simulink model "controle_kanayama"  (R2018a)
settings: Solver=VariableStepAuto  StartTime=0.0  StopTime=7  RelTol=1e-3
values from neighbouring files (symbols this model uses):
  KIm = Pm*KPm    (= 0.759312111233)    [LineFollower.m]    (also in malha_fechada.m)
  Km = 455.5    [LineFollower.m]    (also in malha_aberta.m; malha_fechada.m)
  KPm = 4/(Km*ts_m)    (= 0.0585437248445)    [LineFollower.m]    (also in malha_fechada.m)
  Kteta = 2*qsi*sqrt(Ky)    [LineFollower.m]
  Kx = 4/Ts_x    (= 80)    [LineFollower.m]
  Ky = (wn/v_r)^2    (= 6400)    [LineFollower.m]
  l = 69e-3    (= 0.069)    [LineFollower.m]    (also in malha_aberta.m; malha_fechada.m)
  Pm = 12.97    [LineFollower.m]    (also in malha_aberta.m; malha_fechada.m)
  Qr = [v_r; w_r]    [LineFollower.m]
  r = 16e-3    (= 0.016)    [LineFollower.m]    (also in kinematic_model.m; malha_aberta.m; malha_fechada.m)
libraries: simulink x6
settings Model: Creator=bruno  LastModifiedBy=bruno

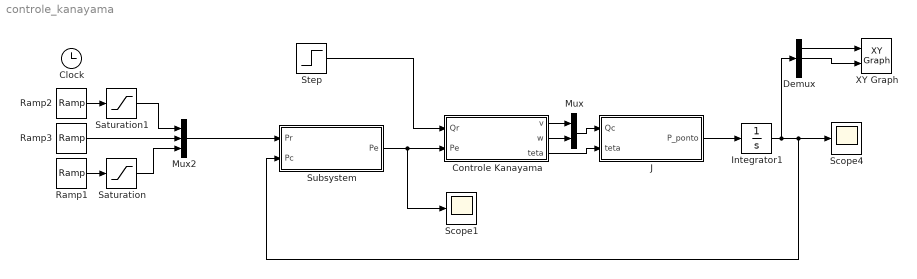
== system controle_kanayama ==
  Clock : Clock
  Controle Kanayama : Subsystem
  Demux : Demux  Outputs=3
  Integrator1 : Integrator
  J : Subsystem
  Mux : Mux  Inputs=2
  Mux2 : Mux  Inputs=3
  Ramp1 : simulink/Sources/Ramp  slope=5  start=0  InitialOutput=0
  Ramp2 : simulink/Sources/Ramp  slope=1  start=0  InitialOutput=0
  Ramp3 : simulink/Sources/Ramp  slope=0  start=0  InitialOutput=0
  Saturation : Saturate  UpperLimit=0
  Saturation1 : Saturate  UpperLimit=1
  Scope1 : Scope
  Scope4 : Scope
  Step : Step  Time=0  After=Qr  SampleTime=0
  Subsystem : Subsystem
  XY Graph : simulink/Sinks/XY Graph  xmin=0  xmax=6  ymin=-0.06  ymax=0.06  st=-1
  wires:
  Integrator1/1 -> Demux/1, Scope4/1, Subsystem/2(Pc)
  Subsystem/1(Pe) -> Scope1/1, Controle Kanayama/2(Pe)
  J/1(P_ponto) -> Integrator1/1
  Mux/1 -> J/1(Qc)
  Controle Kanayama/1(v) -> Mux/1
  Controle Kanayama/2(w) -> Mux/2
  Controle Kanayama/3(teta) -> J/2(teta)
  Step/1 -> Controle Kanayama/1(Qr)
  Ramp3/1 -> Mux2/2
  Ramp1/1 -> Saturation/1
  Saturation/1 -> Mux2/3
  Demux/1 -> XY Graph/1
  Demux/2 -> XY Graph/2
  Ramp2/1 -> Saturation1/1
  Saturation1/1 -> Mux2/1
  Mux2/1 -> Subsystem/1(Pr)

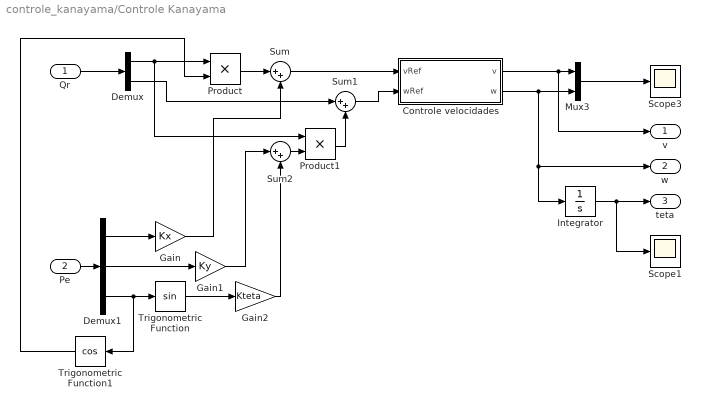
== system controle_kanayama/Controle Kanayama ==
  Qr : Inport
  Pe : Inport  Port=2
  Controle velocidades : Subsystem
  Demux : Demux  Outputs=2
  Demux1 : Demux  Outputs=3
  Gain : Gain  Gain=Kx
  Gain1 : Gain  Gain=Ky
  Gain2 : Gain  Gain=Kteta
  Integrator : Integrator
  Mux3 : Mux  Inputs=2
  Product : Product
  Product1 : Product
  Scope1 : Scope
  Scope3 : Scope
  Sum : Sum  Inputs=|++
  Sum1 : Sum  Inputs=|++
  Sum2 : Sum  Inputs=|++
  Trigonometric Function : Trigonometry
  Trigonometric Function1 : Trigonometry  Operator=cos
  v : Outport
  w : Outport  Port=2
  teta : Outport  Port=3
  wires:
  Controle velocidades/2(w) -> Integrator/1, w/1, Mux3/2
  Controle velocidades/1(v) -> v/1, Mux3/1
  Mux3/1 -> Scope3/1
  Integrator/1 -> Scope1/1, teta/1
  Qr/1 -> Demux/1
  Pe/1 -> Demux1/1
  Demux/1 -> Product/1, Product1/1
  Trigonometric Function/1 -> Gain2/1
  Demux1/3 -> Trigonometric Function1/1, Trigonometric Function/1
  Product/1 -> Sum/1
  Sum/1 -> Controle velocidades/1(vRef)
  Demux1/1 -> Gain/1
  Gain/1 -> Sum/2
  Demux/2 -> Sum1/1
  Product1/1 -> Sum1/2
  Sum1/1 -> Controle velocidades/2(wRef)
  Sum2/1 -> Product1/2
  Demux1/2 -> Gain1/1
  Gain1/1 -> Sum2/1
  Gain2/1 -> Sum2/2
  Trigonometric Function1/1 -> Product/2

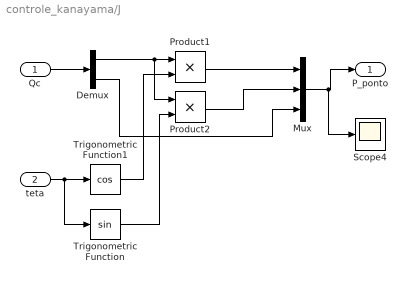
== system controle_kanayama/J ==
  Qc : Inport
  teta : Inport  Port=2
  Demux : Demux  Outputs=2
  Mux : Mux  Inputs=3
  Product1 : Product
  Product2 : Product
  Scope4 : Scope
  Trigonometric Function : Trigonometry
  Trigonometric Function1 : Trigonometry  Operator=cos
  P_ponto : Outport
  wires:
  Mux/1 -> Scope4/1, P_ponto/1
  Qc/1 -> Demux/1
  teta/1 -> Trigonometric Function/1, Trigonometric Function1/1
  Trigonometric Function1/1 -> Product1/2
  Demux/1 -> Product2/1, Product1/1
  Product1/1 -> Mux/1
  Trigonometric Function/1 -> Product2/2
  Product2/1 -> Mux/2
  Demux/2 -> Mux/3

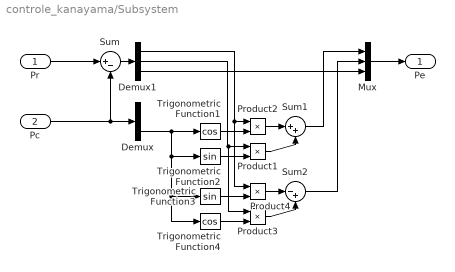
== system controle_kanayama/Subsystem ==
  Pr : Inport
  Pc : Inport  Port=2
  Demux : Demux  Outputs=3
  Demux1 : Demux  Outputs=3
  Mux : Mux  Inputs=3
  Product{1..4} (4 alike) : Product
  Sum : Sum  Inputs=|+-
  Sum1 : Sum  Inputs=|++
  Sum2 : Sum  Inputs=|-+
  Trigonometric Function1 : Trigonometry  Operator=cos
  Trigonometric Function2 : Trigonometry
  Trigonometric Function3 : Trigonometry
  Trigonometric Function4 : Trigonometry  Operator=cos
  Pe : Outport
  wires:
  Pr/1 -> Sum/1
  Pc/1 -> Demux/1, Sum/2
  Demux/3 -> Trigonometric Function4/1, Trigonometric Function3/1, Trigonometric Function2/1, Trigonometric Function1/1
  Sum/1 -> Demux1/1
  Trigonometric Function1/1 -> Product2/2
  Trigonometric Function2/1 -> Product1/2
  Demux1/1 -> Product4/1, Product2/1
  Demux1/2 -> Product3/1, Product1/1
  Product2/1 -> Sum1/1
  Product1/1 -> Sum1/2
  Mux/1 -> Pe/1
  Sum1/1 -> Mux/1
  Trigonometric Function3/1 -> Product4/2
  Product3/1 -> Sum2/2
  Trigonometric Function4/1 -> Product3/2
  Product4/1 -> Sum2/1
  Sum2/1 -> Mux/2
  Demux1/3 -> Mux/3

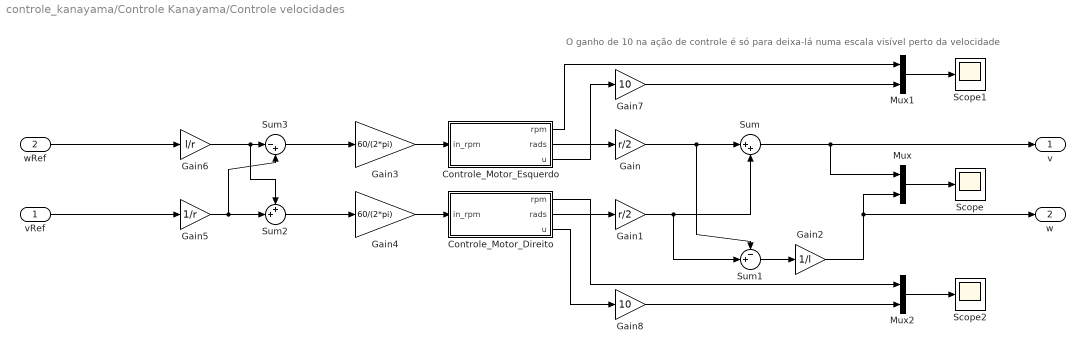
== system controle_kanayama/Controle Kanayama/Controle velocidades ==
  note: O ganho de 10 na ação de controle é só para deixa-lá numa escala visível perto da velocidade
  vRef : Inport
  wRef : Inport  Port=2
  Controle_Motor_Direito : Subsystem
  Controle_Motor_Esquerdo : Subsystem
  Gain : Gain  Gain=r/2
  Gain1 : Gain  Gain=r/2
  Gain2 : Gain  Gain=1/l
  Gain3 : Gain  Gain=60/(2*pi)
  Gain4 : Gain  Gain=60/(2*pi)
  Gain5 : Gain  Gain=1/r
  Gain6 : Gain  Gain=l/r
  Gain7 : Gain  Gain=10
  Gain8 : Gain  Gain=10
  Mux : Mux  Inputs=2
  Mux1 : Mux  Inputs=2
  Mux2 : Mux  Inputs=2
  Scope : Scope
  Scope1 : Scope
  Scope2 : Scope
  Sum : Sum  Inputs=|++
  Sum1 : Sum  Inputs=-+|
  Sum2 : Sum  Inputs=++|
  Sum3 : Sum  Inputs=|-+
  v : Outport
  w : Outport  Port=2
  wires:
  Sum2/1 -> Gain4/1
  vRef/1 -> Gain5/1
  Gain7/1 -> Mux1/2
  wRef/1 -> Gain6/1
  Gain2/1 -> w/1, Mux/2
  Gain1/1 -> Sum1/2, Sum/2
  Sum1/1 -> Gain2/1
  Controle_Motor_Direito/2(rads) -> Gain1/1
  Mux2/1 -> Scope2/1
  Gain3/1 -> Controle_Motor_Esquerdo/1(in_rpm)
  Mux/1 -> Scope/1
  Gain4/1 -> Controle_Motor_Direito/1(in_rpm)
  Gain/1 -> Sum1/1, Sum/1
  Gain5/1 -> Sum2/2, Sum3/2
  Mux1/1 -> Scope1/1
  Gain8/1 -> Mux2/2
  Controle_Motor_Esquerdo/3(u) -> Gain7/1
  Gain6/1 -> Sum2/1, Sum3/1
  Sum3/1 -> Gain3/1
  Controle_Motor_Esquerdo/1(rpm) -> Mux1/1
  Controle_Motor_Direito/3(u) -> Gain8/1
  Sum/1 -> v/1, Mux/1
  Controle_Motor_Direito/1(rpm) -> Mux2/1
  Controle_Motor_Esquerdo/2(rads) -> Gain/1

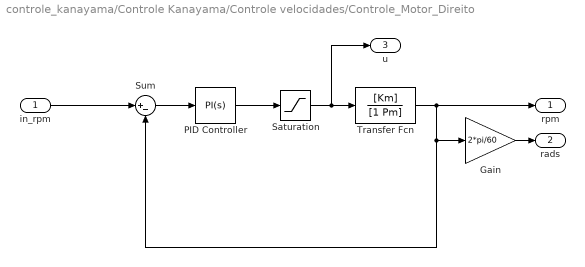
== system controle_kanayama/Controle Kanayama/Controle velocidades/Controle_Motor_Direito ==
  in_rpm : Inport
  Gain : Gain  Gain=2*pi/60
  PID Controller : simulink/Continuous/PID Controller  Controller=PI  TimeDomain=Continuous-time  SampleTime=-1  IntegratorMethod=Forward Euler  FilterMethod=Forward Euler  Form=Parallel  UseFilter=on  ControllerParametersSource=internal  P=KPm  I=KIm  D=0  N=0  InitialConditionSource=internal  InitialConditionForIntegrator=0  InitialConditionForFilter=0  ExternalReset=none  LimitOutput=off  UpperSaturationLimit=inf  LowerSaturationLimit=-inf  LinearizeAsGain=on  AntiWindupMode=none  Kb=1  TrackingMode=off  Kt=1  PParamMin=[]  PParamMax=[]  IParamMin=[]  IParamMax=[]  DParamMin=[]  DParamMax=[]  NParamMin=[]  NParamMax=[]  KbParamMin=[]  KbParamMax=[]  KtParamMin=[]  KtParamMax=[]  POutMin=[]  POutMax=[]  IOutMin=[]  IOutMax=[]  DOutMin=[]  DOutMax=[]  NOutMin=[]  NOutMax=[]  KbOutMin=[]  KbOutMax=[]  KtOutMin=[]  KtOutMax=[]  IntegratorOutMin=[]  IntegratorOutMax=[]  FilterOutMin=[]  FilterOutMax=[]  SumOutMin=[]  SumOutMax=[]  SumI1OutMin=[]  SumI1OutMax=[]  SumI2OutMin=[]  SumI2OutMax=[]  SumI3OutMin=[]  SumI3OutMax=[]  SumDOutMin=[]  SumDOutMax=[]  SaturationOutMin=[]  SaturationOutMax=[]  IntegratorContinuousStateAttributes=''  IntegratorStateMustResolveToSignalObject=off  IntegratorRTWStateStorageClass=Auto  FilterContinuousStateAttributes=''  FilterStateMustResolveToSignalObject=off  FilterRTWStateStorageClass=Auto  DifferentiatorICPrevScaledInput=0  DifferentiatorOutMin=[]  DifferentiatorOutMax=[]  FilterDiffOutCoefMin=[]  FilterDiffOutCoefMax=[]  SumDenOutMin=[]  SumDenOutMax=[]  SumNumOutMin=[]  SumNumOutMax=[]  ReciprocalOutMin=[]  ReciprocalOutMax=[]  DivideOutMin=[]  DivideOutMax=[]  TunerSelectOption=Transfer Function Based (PID Tuner App)
  Saturation : Saturate  UpperLimit=100  LowerLimit=-100
  Sum : Sum  Inputs=|+-
  Transfer Fcn : TransferFcn  Numerator=[Km]  Denominator=[1 Pm]
  rpm : Outport
  rads : Outport  Port=2
  u : Outport  Port=3
  wires:
  PID Controller/1 -> Saturation/1
  Transfer Fcn/1 -> rpm/1, Gain/1, Sum/2
  Saturation/1 -> u/1, Transfer Fcn/1
  Sum/1 -> PID Controller/1
  in_rpm/1 -> Sum/1
  Gain/1 -> rads/1

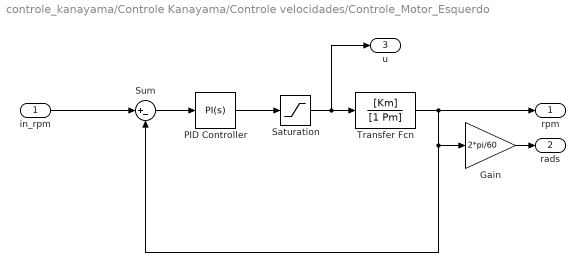
== system controle_kanayama/Controle Kanayama/Controle velocidades/Controle_Motor_Esquerdo ==
  in_rpm : Inport
  Gain : Gain  Gain=2*pi/60
  PID Controller : simulink/Continuous/PID Controller  Controller=PI  TimeDomain=Continuous-time  SampleTime=-1  IntegratorMethod=Forward Euler  FilterMethod=Forward Euler  Form=Parallel  UseFilter=on  ControllerParametersSource=internal  P=KPm  I=KIm  D=0  N=0  InitialConditionSource=internal  InitialConditionForIntegrator=0  InitialConditionForFilter=0  ExternalReset=none  LimitOutput=off  UpperSaturationLimit=inf  LowerSaturationLimit=-inf  LinearizeAsGain=on  AntiWindupMode=none  Kb=1  TrackingMode=off  Kt=1  PParamMin=[]  PParamMax=[]  IParamMin=[]  IParamMax=[]  DParamMin=[]  DParamMax=[]  NParamMin=[]  NParamMax=[]  KbParamMin=[]  KbParamMax=[]  KtParamMin=[]  KtParamMax=[]  POutMin=[]  POutMax=[]  IOutMin=[]  IOutMax=[]  DOutMin=[]  DOutMax=[]  NOutMin=[]  NOutMax=[]  KbOutMin=[]  KbOutMax=[]  KtOutMin=[]  KtOutMax=[]  IntegratorOutMin=[]  IntegratorOutMax=[]  FilterOutMin=[]  FilterOutMax=[]  SumOutMin=[]  SumOutMax=[]  SumI1OutMin=[]  SumI1OutMax=[]  SumI2OutMin=[]  SumI2OutMax=[]  SumI3OutMin=[]  SumI3OutMax=[]  SumDOutMin=[]  SumDOutMax=[]  SaturationOutMin=[]  SaturationOutMax=[]  IntegratorContinuousStateAttributes=''  IntegratorStateMustResolveToSignalObject=off  IntegratorRTWStateStorageClass=Auto  FilterContinuousStateAttributes=''  FilterStateMustResolveToSignalObject=off  FilterRTWStateStorageClass=Auto  DifferentiatorICPrevScaledInput=0  DifferentiatorOutMin=[]  DifferentiatorOutMax=[]  FilterDiffOutCoefMin=[]  FilterDiffOutCoefMax=[]  SumDenOutMin=[]  SumDenOutMax=[]  SumNumOutMin=[]  SumNumOutMax=[]  ReciprocalOutMin=[]  ReciprocalOutMax=[]  DivideOutMin=[]  DivideOutMax=[]  TunerSelectOption=Transfer Function Based (PID Tuner App)
  Saturation : Saturate  UpperLimit=100  LowerLimit=-100
  Sum : Sum  Inputs=|+-
  Transfer Fcn : TransferFcn  Numerator=[Km]  Denominator=[1 Pm]
  rpm : Outport
  rads : Outport  Port=2
  u : Outport  Port=3
  wires:
  PID Controller/1 -> Saturation/1
  Saturation/1 -> u/1, Transfer Fcn/1
  Sum/1 -> PID Controller/1
  in_rpm/1 -> Sum/1
  Transfer Fcn/1 -> rpm/1, Gain/1, Sum/2
  Gain/1 -> rads/1
